simulink model "threephinv"  (R2015a)
settings: Solver=ode23tb  StartTime=0.0  StopTime=1  RelTol=1e-3
libraries: powerlib x25, simulink x3, powerlib_meascontrol x1
settings Model: Creator=Ratish Kumar S  LastModifiedBy=Ratish Kumar S

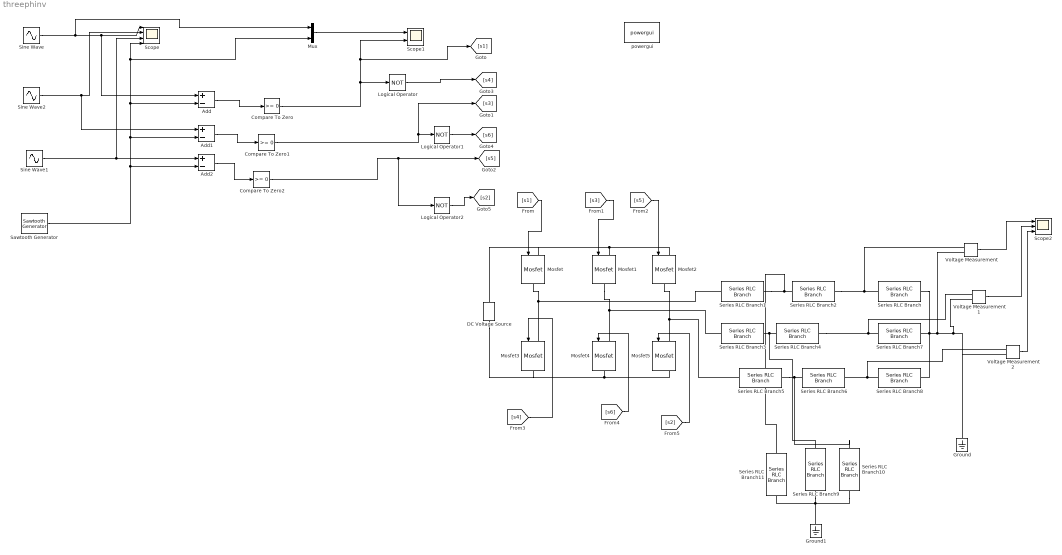
== system threephinv ==
  Add : Sum  Inputs=+-
  Add1 : Sum  Inputs=+-
  Add2 : Sum  Inputs=+-
  Compare To Zero : simulink/Logic and Bit Operations/Compare To Zero  relop=>=  OutDataTypeStr=boolean
  Compare To Zero1 : simulink/Logic and Bit Operations/Compare To Zero  relop=>=  OutDataTypeStr=boolean
  Compare To Zero2 : simulink/Logic and Bit Operations/Compare To Zero  relop=>=  OutDataTypeStr=boolean
  DC Voltage Source : powerlib/Electrical Sources/DC Voltage Source  Amplitude=170  Measurements=None
  Ground : powerlib/Elements/Ground  LConnTagsString=a
  Ground1 : powerlib/Elements/Ground  LConnTagsString=a
  Logical Operator : Logic  Operator=NOT  AllPortsSameDT=off  OutDataTypeStr=boolean
  Logical Operator1 : Logic  Operator=NOT  AllPortsSameDT=off  OutDataTypeStr=boolean
  Logical Operator2 : Logic  Operator=NOT  AllPortsSameDT=off  OutDataTypeStr=boolean
  Mosfet{,1..4} (5 alike) : powerlib/Power Electronics/Mosfet  Ron=0.1  Lon=0  Rd=0.01  Vfd=0  IC=0  Rs=1e5  Cs=inf  Measurements=off
  Mosfet5 : powerlib/Power Electronics/Mosfet  Ron=0.1  Lon=0  Rd=0.01  Vfd=0  IC=0  Rs=1e5  Cs=inf  Measurements=on
  Mux : Mux  Inputs=2
  Sawtooth Generator : powerlib_meascontrol/Pulse & Signal Generators/Sawtooth Generator  Freq=1e3  Phase=180  Ts=0
  Scope : Scope  NumInputPorts=4
      settings: YMin=-5~-5~-5~-5  YMax=5~5~5~5
  Scope1 : Scope  NumInputPorts=2
      settings: YMin=-5~-5  YMax=5~5
  Scope2 : Scope  NumInputPorts=3
      settings: YMin=-80~-80~-80  YMax=90~90~80  SaveName=ScopeData2
  Series RLC Branch : powerlib/Elements/Series RLC Branch  LConnTagsString=__new0  RConnTagsString=__new0  BranchType=R  Resistance=1e5  Inductance=1e-3  SetiL0=off  InitialCurrent=0  Capacitance=1e-2  Setx0=off  InitialVoltage=0  Measurements=None
  Series RLC Branch{1..6} (6 alike) : powerlib/Elements/Series RLC Branch  LConnTagsString=__new0  RConnTagsString=__new0  BranchType=L  Resistance=1e5  Inductance=1e-3  SetiL0=off  InitialCurrent=0  Capacitance=1e-2  Setx0=off  InitialVoltage=0  Measurements=None
  Series RLC Branch10 : powerlib/Elements/Series RLC Branch  LConnTagsString=__new0  RConnTagsString=__new0  BranchType=C  Resistance=1e5  Inductance=1e-3  SetiL0=off  InitialCurrent=0  Capacitance=1e-2  Setx0=off  InitialVoltage=0  Measurements=None
  Series RLC Branch11 : powerlib/Elements/Series RLC Branch  LConnTagsString=__new0  RConnTagsString=__new0  BranchType=C  Resistance=1e5  Inductance=1e-3  SetiL0=off  InitialCurrent=0  Capacitance=1e-2  Setx0=off  InitialVoltage=0  Measurements=None
  Series RLC Branch7 : powerlib/Elements/Series RLC Branch  LConnTagsString=__new0  RConnTagsString=__new0  BranchType=R  Resistance=1e5  Inductance=1e-3  SetiL0=off  InitialCurrent=0  Capacitance=1e-2  Setx0=off  InitialVoltage=0  Measurements=None
  Series RLC Branch8 : powerlib/Elements/Series RLC Branch  LConnTagsString=__new0  RConnTagsString=__new0  BranchType=R  Resistance=1e5  Inductance=1e-3  SetiL0=off  InitialCurrent=0  Capacitance=1e-2  Setx0=off  InitialVoltage=0  Measurements=None
  Series RLC Branch9 : powerlib/Elements/Series RLC Branch  LConnTagsString=__new0  RConnTagsString=__new0  BranchType=C  Resistance=1e5  Inductance=1e-3  SetiL0=off  InitialCurrent=0  Capacitance=1e-2  Setx0=off  InitialVoltage=0  Measurements=None
  Sine Wave : Sin  Frequency=2*pi*50  SampleTime=0
  Sine Wave1 : Sin  Frequency=2*pi*50  Phase=-2*pi/3  SampleTime=0
  Sine Wave2 : Sin  Frequency=2*pi*50  Phase=2*pi/3  SampleTime=0
  Voltage Measurement : powerlib/Measurements/Voltage Measurement  PhasorSimulation=off  OutputType=Complex  PSBequivalent=0
  Voltage Measurement1 : powerlib/Measurements/Voltage Measurement  PhasorSimulation=off  OutputType=Complex  PSBequivalent=0
  Voltage Measurement2 : powerlib/Measurements/Voltage Measurement  PhasorSimulation=off  OutputType=Complex  PSBequivalent=0
  powergui : powerlib/powergui  Priority=1  SimulationMode=Continuous  SolverType=Tustin/Backward Euler (TBE)  SampleTime=50e-6  frequency=60  SPID=off  DisableSnubberDevices=off  DisableRonSwitches=off  DisableVfSwitches=off  SwTol=0  DisplayEquations=off  Interpol=off  methode=off  Ts=100  FunctionMessages=off  echomessages=off  HookPort=off  EnableUseOfTLC=off  x0status=blocks  frequencyindice=0  Pbase=100e6  ErrMax=1e-4  Iterations=50  UnitsV=kV  UnitsW=MW  buscounter=0  RestoreLinks=warning  ResistiveCurrentMeasurement=off  Frange=[0:2:500]  Ylog=off  Xlog=on  ShowGrid=off  save=off  variable=ZData  structure=0  ZoomFFT=off  StartTime=0.0  cycles=1  DisplayStyle=1  fundamental=60  FreqAxis=off  MaxFrequency=1000  frequencyindicesteady=1  RmsSteady=1  display=off
  wires:
  Sine Wave1/1 -> Add2/1, Scope/3
  Sine Wave/1 -> Mux/1, Add/1, Scope/1
  Sine Wave2/1 -> Add1/1, Scope/2
  Sawtooth Generator/1 -> Add2/2, Add/2, Mux/2, Scope/4, Add1/2
  Add/1 -> Compare To Zero/1
  Add1/1 -> Compare To Zero1/1
  Add2/1 -> Compare To Zero2/1
  Mux/1 -> Scope1/1
  Compare To Zero/1 -> Logical Operator/1, [s1], Scope1/2
  Compare To Zero1/1 -> Logical Operator1/1, [s3]
  Compare To Zero2/1 -> Logical Operator2/1, [s5]
  Logical Operator/1 -> [s4]
  Logical Operator1/1 -> [s6]
  Logical Operator2/1 -> [s2]
  [s1] -> Mosfet/1
  [s3] -> Mosfet1/1
  [s5] -> Mosfet2/1
  [s4] -> Mosfet3/1
  [s6] -> Mosfet4/1
  [s2] -> Mosfet5/1
  Voltage Measurement/1 -> Scope2/1
  Voltage Measurement1/1 -> Scope2/2
  Voltage Measurement2/1 -> Scope2/3
  connections:
  Mosfet/RConn1 -- Series RLC Branch1/LConn1 -- Mosfet3/LConn1
  Mosfet1/RConn1 -- Series RLC Branch3/LConn1 -- Mosfet4/LConn1
  Mosfet2/RConn1 -- Series RLC Branch5/LConn1 -- Mosfet5/LConn1
  Mosfet4/RConn1 -- Mosfet5/RConn1 -- DC Voltage Source/LConn1 -- Mosfet3/RConn1
  Mosfet1/LConn1 -- DC Voltage Source/RConn1 -- Mosfet/LConn1 -- Mosfet2/LConn1
  Series RLC Branch1/RConn1 -- Series RLC Branch11/LConn1 -- Series RLC Branch2/LConn1
  Series RLC Branch2/RConn1 -- Voltage Measurement/LConn1 -- Series RLC Branch/LConn1
  Series RLC Branch4/LConn1 -- Series RLC Branch9/LConn1 -- Series RLC Branch3/RConn1
  Series RLC Branch4/RConn1 -- Voltage Measurement1/LConn1 -- Series RLC Branch7/LConn1
  Series RLC Branch5/RConn1 -- Series RLC Branch10/LConn1 -- Series RLC Branch6/LConn1
  Series RLC Branch8/LConn1 -- Voltage Measurement2/LConn1 -- Series RLC Branch6/RConn1
  Series RLC Branch/RConn1 -- Voltage Measurement2/LConn2 -- Ground/LConn1 -- Voltage Measurement1/LConn2 -- Voltage Measurement/LConn2 -- Series RLC Branch7/RConn1 -- Series RLC Branch8/RConn1
  Series RLC Branch10/RConn1 -- Ground1/LConn1 -- Series RLC Branch9/RConn1 -- Series RLC Branch11/RConn1
